simulink model "sl_model_function_2016"  (R2016b)
settings: Solver=VariableStepAuto  StartTime=0.0  StopTime=10.0  RelTol=1e-3
values from neighbouring files (symbols this model uses):
  x_op_linearise = [pi; 0; pi; 0]    [LQR_main.m]
settings Model: Creator=jonathan  LastModifiedBy=jkleinschiphor
settings SFSimCC: SimUseLocalCustomCode=on
settings RTWCC: RTWUseLocalCustomCode=on

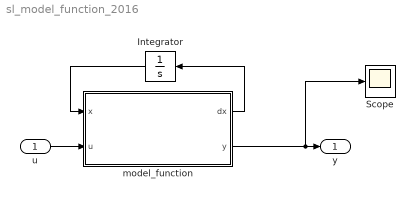
== system sl_model_function_2016 ==
  u : Inport
  Integrator : Integrator  InitialCondition=x_op_linearise
  Scope : Scope
  model_function : MATLAB Function  TreatAsAtomicUnit=on
  y : Outport
  wires:
  model_function/1(dx) -> Integrator/1
  u/1 -> model_function/2(u)
  Integrator/1 -> model_function/1(x)
  model_function/2(y) -> y/1, Scope/1

== matlab function sl_model_function_2016/model_function ==
  data: dx output; y output; x input; u input
function [dx, y] = model_function(x, u)
g = 9.81;

m1 = 0.125;
c1 = 0.06;
L1 = 0.1;
I1 = 0.074;

m2 = 0.05;
c2 = 0.06;
L2 = 0.1;
I2 = 0.00012;

Beta1 = 4.8;
Beta2 = 0.0002;
Ki = 50;
tau_e = 0.03;

P1 = m1*c1^2 + m2*L1^2 + I1;
P2 = m2*c2^2 + I2;
P3 = m2*L1*c2;
g1 = (m1*c1 + m2*L1)*g;
g2 = m2*c2*g;


M = [P1+P2+2*P3*cos(x(3)) P2+P3*cos(x(3)) ; ...
     P2 + P3*cos(x(3))    P2];
 
C = [Beta1 - P3*x(4)*sin(x(3)) -P3*(x(2)+x(4))*sin(x(3)); ...
     P3*x(2)*sin(x(3))         Beta2];
 
G = [-g1*sin(x(1)) - g2*sin(x(1)+x(3)); ...
     -g2*sin(x(1)+x(3))];
Minv = inv(M);

th_dd = Minv*[Ki*u; 0] - Minv*C*[x(2) ; x(4)] - Minv*G;

dx = [x(2); ...
      th_dd(1); ...
      x(4); ...
      th_dd(2)];
  
y = [1 0 0 0; 0 0 1 0]*x;

end
